simulink library "Inverter"  (Simulink 8.2)
settings: Solver=ode45  StartTime=0.0  StopTime=10.0  RelTol=1e-3
settings Model: Creator=lena.frank  LastModifiedBy=drhf

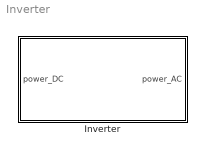
== system Inverter ==
  Inverter : Subsystem  mask(Inverter_simple){P0=9000, ol=1.2, power_steps=[0 0.05 0.1 0.2 0.3 0.5 1 1.2], eta_steps=[0 0.924 0.958 0.974 0.979 0.981 0.98 0.95], standby=0}
      mask prompts: P0 "nominal power"; ol "overload (0.5 ...1.5)"; power_steps "steps for efficiency (0..1..overload)"; eta_steps "efficiency (0..1)"; standby "Standby power consumption in W"
      mask help:
      | This block considers the eficiency of the inverter based on
      | - eta euro [1]
      |
      | In the simple model the efficieny of the inverter is assumed to be constant.
      mask Help: web(fullfile(path_carnot('help'),'Inverter.html'),'-helpbrowser')
      mask Display:
      | %plot([0,0],[0,1],[-0.5,1.5],[0,0],power_steps, eta_steps)
      | plot(-40,0,140,100,[90,10,90,90,10,10],[10,90,90,10,10,90],[40,20],[40,40],[40,20],[30,30],[88,84,75,64,55,50],[70,60,60,80,80,70])

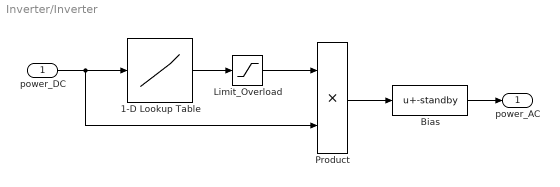
== system Inverter/Inverter ==
  power_DC : Inport
  1-D Lookup Table : Lookup_n-D  NumberOfTableDimensions=1  BreakpointsForDimension1=power_steps*P0  Table=eta_steps  RndMeth=Simplest  InputSameDT=on
  Bias : Bias  Bias=-standby
  Limit_Overload : Saturate  UpperLimit=ol  LowerLimit=0
  Product : Product
  power_AC : Outport
  wires:
  power_DC/1 -> Product/2, 1-D Lookup Table/1
  1-D Lookup Table/1 -> Limit_Overload/1
  Limit_Overload/1 -> Product/1
  Product/1 -> Bias/1
  Bias/1 -> power_AC/1
